simulink model "Feedback_Lin_MECC2025"  (R2021a)
settings: Solver=ode1  StartTime=0.0  StopTime=50  FixedStep=1e-3  RelTol=1e-3
values from neighbouring files (symbols this model uses):
  x0 = 4.*[1, 3, 0.05]    [sim_main_script_newparams.m]
settings Model: Creator=g.liu1  LastModifiedBy=Amanda
settings DebuggingCC: UnconnectedInputMsg=none  UnconnectedOutputMsg=none  UnconnectedLineMsg=none
settings ModelReferenceCC: EnableRefExpFcnMdlSchedulingChecks=off
settings RTWCC: Description=Generic Real-Time Target  DLArmComputeVersion=20.02.1

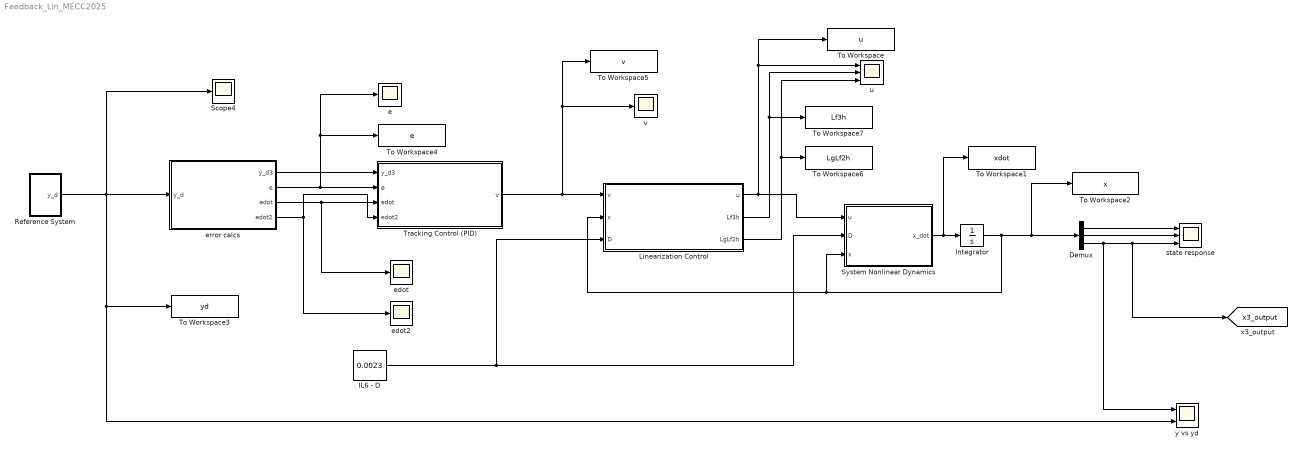
== system Feedback_Lin_MECC2025 ==
  Demux : Demux  Outputs=3
  IL6 - D : Constant  Value=0.0023
  Integrator : Integrator  InitialCondition=x0
  Linearization Control : MATLAB Function  TreatAsAtomicUnit=on
  Reference System : Subsystem
  Scope4 : Scope
  System Nonlinear Dynamics : MATLAB Function  TreatAsAtomicUnit=on
  To Workspace : ToWorkspace  VariableName=u  SaveFormat=Timeseries  SampleTime=-1
  To Workspace1 : ToWorkspace  VariableName=xdot  SaveFormat=Timeseries  SampleTime=-1
  To Workspace2 : ToWorkspace  VariableName=x  SaveFormat=Timeseries  SampleTime=-1
  To Workspace3 : ToWorkspace  VariableName=yd  SaveFormat=Timeseries  SampleTime=-1
  To Workspace4 : ToWorkspace  VariableName=e  SaveFormat=Timeseries  SampleTime=-1
  To Workspace5 : ToWorkspace  VariableName=v  SaveFormat=Timeseries  SampleTime=-1
  To Workspace6 : ToWorkspace  VariableName=LgLf2h  SaveFormat=Timeseries  SampleTime=-1
  To Workspace7 : ToWorkspace  VariableName=Lf3h  SaveFormat=Timeseries  SampleTime=-1
  Tracking Control (PID) : MATLAB Function  TreatAsAtomicUnit=on
  e : Scope
  edot : Scope
  edot2 : Scope
  error calcs : Subsystem
  state response : Scope  NumInputPorts=3
  u : Scope  NumInputPorts=3
  v : Scope
  y vs yd : Scope  NumInputPorts=2
  tag scope: x3_output=global
  wires:
  Reference System/1(y_d) -> error calcs/1(y_d), Scope4/1, y vs yd/2, To Workspace3/1
  error calcs/1(y_d3) -> Tracking Control (PID)/1(y_d3)
  error calcs/2(e) -> To Workspace4/1, e/1, Tracking Control (PID)/2(e)
  error calcs/3(edot) -> edot/1, Tracking Control (PID)/3(edot)
  error calcs/4(edot2) -> edot2/1, Tracking Control (PID)/4(edot2)
  Tracking Control (PID)/1(v) -> To Workspace5/1, v/1, Linearization Control/1(v)
  Linearization Control/1(u) -> System Nonlinear Dynamics/1(u), To Workspace/1, u/1
  IL6 - D/1 -> System Nonlinear Dynamics/2(D), Linearization Control/3(D)
  System Nonlinear Dynamics/1(x_dot) -> To Workspace1/1, Integrator/1
  Integrator/1 -> To Workspace2/1, Demux/1, Linearization Control/2(x), System Nonlinear Dynamics/3(x)
  Demux/1 -> state response/1
  Demux/2 -> state response/2
  Demux/3 -> y vs yd/1, [x3_output], state response/3
  Linearization Control/2(Lf3h) -> u/2, To Workspace7/1
  Linearization Control/3(LgLf2h) -> u/3, To Workspace6/1

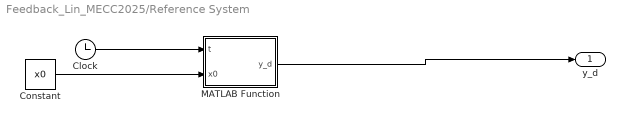
== system Feedback_Lin_MECC2025/Reference System ==
  Clock : Clock
  Constant : Constant  Value=x0
  MATLAB Function : MATLAB Function  TreatAsAtomicUnit=on
  y_d : Outport
  wires:
  Clock/1 -> MATLAB Function/1(t)
  MATLAB Function/1(y_d) -> y_d/1
  Constant/1 -> MATLAB Function/2(x0)

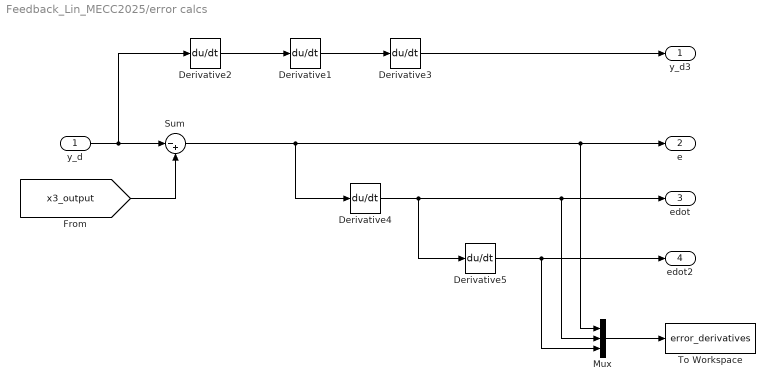
== system Feedback_Lin_MECC2025/error calcs ==
  y_d : Inport
  Derivative{1..5} (5 alike) : Derivative  CoefficientInTFapproximation=0
  Mux : Mux  Inputs=3
  Sum : Sum  Inputs=|-+
  To Workspace : ToWorkspace  VariableName=error_derivatives  SaveFormat=Timeseries  SampleTime=-1
  y_d3 : Outport
  e : Outport  Port=2
  edot : Outport  Port=3
  edot2 : Outport  Port=4
  wires:
  Sum/1 -> Derivative4/1, Mux/1, e/1
  y_d/1 -> Derivative2/1, Sum/1
  [x3_output] -> Sum/2
  Derivative2/1 -> Derivative1/1
  Derivative1/1 -> Derivative3/1
  Derivative3/1 -> y_d3/1
  Derivative4/1 -> Derivative5/1, Mux/2, edot/1
  Derivative5/1 -> Mux/3, edot2/1
  Mux/1 -> To Workspace/1

== matlab function Feedback_Lin_MECC2025/Linearization Control ==
  data: v input; u output; x input; D input; Lf3h output; LgLf2h output
function [u, Lf3h, LgLf2h] = LinearizationControl(v, x, D)
% this function linearizes the nonlinear dynamics 

z1 = 0.8;  % 1/ nM min      -- activation/upregulation of Xa_Va by Fbn 
g1 = 10;   % 1/min      -- upregulation of Xa_Va by IL6
a1 = 1;    % 1/nM min   -- downregulation by APC input and Xa_Va 
d1 = 0.12; % 1/min      -- natural degradation of Xa_Va -- based on HM for prothrombinase 
K2 = 0.034 * log(2)/4; % equals 0.0059;  % nM/min     -- natural production of tPA
a2 = 15;   % 1/nM min   -- downregulation by IL6 and tPA
n2 = 1.5;  % 1/nM min   -- upregulation by APC input and tPA
z2 = 0.5;  % 1/nM min 
d2 = log(2)/4; % equals 0.1733;  % 1/min      -- natural degradation of tPA 
g3 = 20;   % 1/min      -- upregulation by Xa_Va
z3 = 0.01; % 1/nM min 
d3 = 0.0046; % 1/min      -- natural degradation of fibrin  

% D1 = 0.0023; % nM 
% D1 = 0; 

% U1 = 0; % no APC input 

x1 = x(1);
x2 = x(2);
x3 = x(3);
h = [0 0 1]; 

% x1_dot = z1*x1*x3 + g1*D - d1*x1 - x1*u; %  z1*x1*x3 + g1*D - d1*x1 - a1*x1*u; 
x2_dot = K2 - a2*D*x2 + n2*x1 - z2*x2*x3 - d2*x2; 
x3_dot = g3*D - z3*x2*x3 - d3*x3;

C1 = d3^2 - z3*K2;
C2 = a2*D*z3 + d2*z3 + 2*d3*z3;

alpha_px = C1*x3_dot + C2*x2_dot*x3 + C2*x2*x3_dot - n2*z3*x1*x3_dot + z1*x2_dot*x3^2 + 2*z1*x2*x3*x3_dot + 2*z3^2*x2*x2_dot*x3 + z3^2*x2^2*x3_dot;
alpha_x = alpha_px - n2*z1*z3*x1*x3^2 - n2*z3*g1*D*x3 + d1*n2*z3*x1*x3;
Lf2h = -z3*n2*x1*x3 - z3*g3*D*x2 + a2*D*z3*x2*x3 + z2*z3*x2*x3^2 + d2*z3*x2*x3 + z3^2*x3*x2^2 + 2* d3*z3*x2*x3 + d3^2*x3 - z3*K2*x3 - d3*g3*D; 

% partial derivatives: 
Lf2h_px1 = -z3*n2*x3; 
Lf2h_px2 = -z3*g3*D + a2*D*z3*x3 + z2*z3*x3^2 + d2*z3*x3 + 2*z3^2*x3*x2 + 2*d3*z3*x3; 
Lf2h_px3 = -z3*n2*x1 + a2*D*z3*x2 + 2*z2*z3*x2*x3 + d2*z3*x2 + z3^2*x2^2 + 2* d3*z3*x2 + d3^2 - z3*K2; 

f = [z1*x1*x3 + g1*D - d1*x1; 
     K2 - a2*D*x2 + n2*x1 - z2*x2*x3 - d2*x2; 
     g3*D - z3*x2*x3 - d3*x3];

Lf3h = [Lf2h_px1, Lf2h_px2, Lf2h_px3] * f;

LgLf2h = a1*z3*n2*x1*x3;  

% u = 1/(LgLf^n-1h(x)) * (-Lf^nh(x) + v); % generic format of linearizing
% input, our n = 3 

% u = v; % use in the case when you just want to check tracking controller
% u = 0; % use when want no linearizing controller 
u = (1/(LgLf2h)) * (-Lf3h + v) ;

== matlab function Feedback_Lin_MECC2025/Tracking Control (PID) ==
  data: y_d3 input; e input; v output; edot input; edot2 input; gain parameter
function v = TrackingControl(y_d3, e, edot, edot2, gain)
% v = yd''' - k3*e'' - k2*e' - k1*e;  % General format of reference
% tracking controller 
v = y_d3 - gain.k3*edot2 - gain.k2*edot - gain.k1*e;
% v = 0; % use when want to turn off reference tracking control

== matlab function Feedback_Lin_MECC2025/System Nonlinear Dynamics ==
  data: u input; D input; x_dot output; x input
function x_dot = NonlinearDynamics(u,D,x)
z1 = 0.8;  % 1/ nM min      -- activation/upregulation of Xa_Va by Fbn 
g1 = 10;   % 1/min      -- upregulation of Xa_Va by IL6
a1 = 1;    % 1/nM min   -- downregulation by APC input and Xa_Va 
d1 = 0.12; % 1/min      -- natural degradation of Xa_Va -- based on HM for prothrombinase 
K2 = 0.034 * log(2)/4; % equals 0.0059;  % nM/min     -- natural production of tPA
a2 = 15;   % 1/nM min   -- downregulation by IL6 and tPA
n2 = 1.5;  % 1/nM min   -- upregulation by APC input and tPA
z2 = 0.5;  % 1/nM min 
d2 = log(2)/4; % equals 0.1733;  % 1/min      -- natural degradation of tPA 
g3 = 20;   % 1/min      -- upregulation by Xa_Va
z3 = 0.01; % 1/nM min 
d3 = 0.0046; % 1/min      -- natural degradation of fibrin  

% D1 = 0.0023; % nM 
% D1 = 0; 

x1 = x(1); 
x2 = x(2); 
x3 = x(3); 

% sys =  [(z1*x1*x3 + g1*D1 - d1*x1 - a1*x1*U1), 
%         (K2 - a2*D1*x2 + n2*x1 - z2*x2*x3 - d2*x2),
%         (g3*D1 - z3*x2*x3 - d3*x3)]; 
    
x1_dot = z1*x1*x3 + g1*D - d1*x1 - a1*x1*u; %  z1*x1*x3 + g1*D - d1*x1 - a1*x1*u; 
x2_dot = K2 - a2*D*x2 + n2*x1 - z2*x2*x3 - d2*x2; 
x3_dot = g3*D - z3*x2*x3 - d3*x3;

x_dot=[x1_dot;x2_dot;x3_dot];

== matlab function Feedback_Lin_MECC2025/Reference System/MATLAB Function ==
  data: t input; y_d output; x0 input
function y_d = fcn(t, x0)
y_d = ref_signal(t, x0);
